simulink model "Unit_Step_Response3B"  (R2021b)
settings: Solver=VariableStepAuto  StartTime=0.0  StopTime=10.0  RelTol=1e-3
settings Model: Creator=Richi  LastModifiedBy=Richi

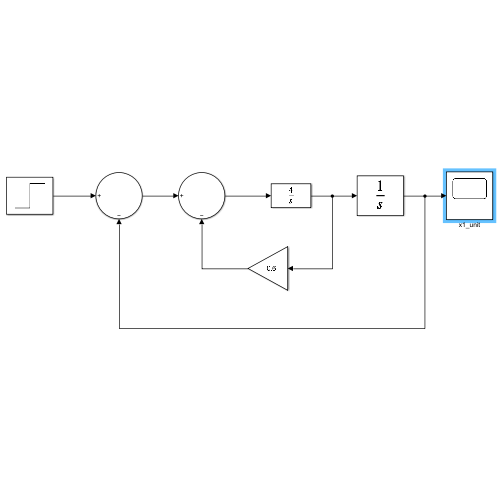
[thumbnail: Simulink's stored preview of the top-level diagram]
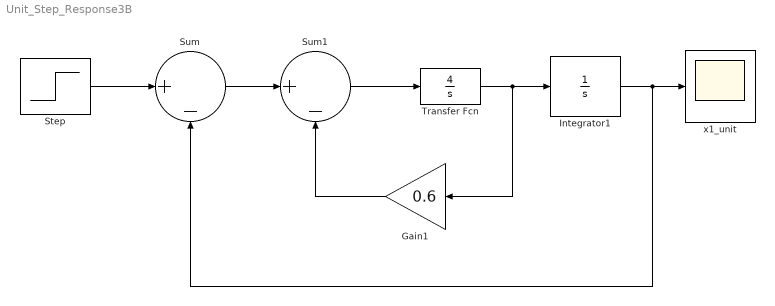
== system Unit_Step_Response3B ==
  Gain1 : Gain  Gain=0.6
  Integrator1 : Integrator
  Step : Step  SampleTime=0
  Sum : Sum  Inputs=|+-
  Sum1 : Sum  Inputs=|+-
  Transfer Fcn : TransferFcn  Numerator=[4]  Denominator=[1 0]
  x1_unit : Scope
  wires:
  Sum/1 -> Sum1/1
  Step/1 -> Sum/1
  Integrator1/1 -> Sum/2, x1_unit/1
  Gain1/1 -> Sum1/2
  Sum1/1 -> Transfer Fcn/1
  Transfer Fcn/1 -> Gain1/1, Integrator1/1
